simulink model "p3"  (R2014b)
settings: Solver=ode45  StartTime=0.0  StopTime=10  RelTol=1e-3
undefined symbols (not defined in the file): fdesignblkfcn, gcbh
settings Model: CovSFcnEnable=on  Creator=dhruv  LastModifiedBy=Kumar
settings OptimizationCC: UseDivisionForNetSlopeComputation=off  SimCompilerOptimization=off
settings DebuggingCC: SolverPrmCheckMsg=none  FrameProcessingCompatibilityMsg=error
settings RTWCC: RTWCompilerOptimization=off

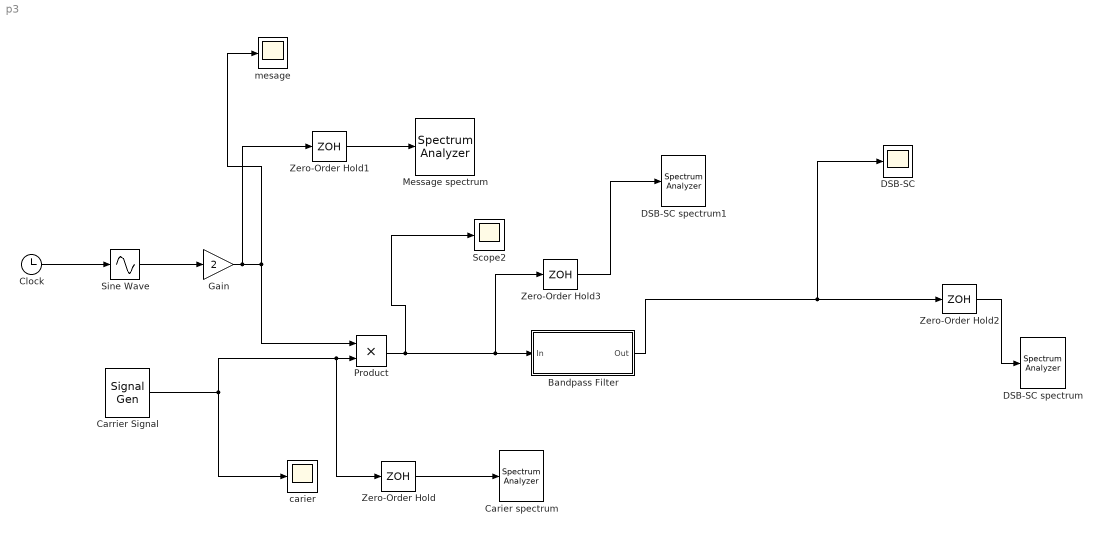
== system p3 ==
  Bandpass Filter : Subsystem  DialogController=fdesignblkfcn  InitFcn=fdesignblkfcn(gcbh, {'InitFcn'});  mask(Bandpass Filter){}
      mask help: Design a bandpass filter
      settings: CopyFcn=fdesignblkfcn(gcbh, {'CopyFcn'});
      mask Help: helpview(mapfilelocation('dsp'), 'dspbandpassfilter');
      mask Display: disp('Bandpass');
  Carier spectrum : SpectrumAnalyzer
  Carrier Signal : SignalGenerator  Frequency=5000
  Clock : Clock
  DSB-SC : Scope
      settings: SaveName=ScopeData4
  DSB-SC spectrum : SpectrumAnalyzer
  DSB-SC spectrum1 : SpectrumAnalyzer
  Gain : Gain  Gain=2
  Message spectrum : SpectrumAnalyzer
  Product : Product
  Scope2 : Scope
      settings: SaveName=ScopeData2
  Sine Wave : Sin  TimeSource=Use external signal  Frequency=2*pi*200  Phase=pi/2  SampleTime=1/4000
  Zero-Order Hold{,1..3} (4 alike) : ZeroOrderHold  SampleTime=1/30000
  carier : Scope
  mesage : Scope
      settings: TickLabels=on  TimeRange=0.05  SampleInput=on
  wires:
  Sine Wave/1 -> Gain/1
  Gain/1 -> Zero-Order Hold1/1, Product/1, mesage/1
  Zero-Order Hold1/1 -> Message spectrum/1
  Zero-Order Hold/1 -> Carier spectrum/1
  Carrier Signal/1 -> Zero-Order Hold/1, Product/2, carier/1
  Zero-Order Hold2/1 -> DSB-SC spectrum/1
  Clock/1 -> Sine Wave/1
  Product/1 -> Bandpass Filter/1(In), Zero-Order Hold3/1, Scope2/1
  Zero-Order Hold3/1 -> DSB-SC spectrum1/1
  Bandpass Filter/1(Out) -> DSB-SC/1, Zero-Order Hold2/1

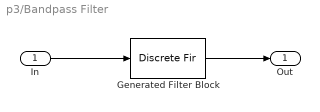
== system p3/Bandpass Filter ==
  In : Inport
  Generated Filter Block : DiscreteFir  Tag=BlockMethodSubSystem  Coefficients=[-4.2089415837660872e-05 -0.0014025699359127397 7.7506550936949734e-05 0.00057128919349381125 -9.8355641636346664e-05 -0.00066711051664750044 0.00015948550574925059 0.00075631980649035072 -0.00023183227068351514 -0.00083532589626739736 0.00031333464421453628 0.00089962011893319322 -0.00040054007469883838 -0.00094474087932631967 0.00048884052624121666 0.00096656259656608529 -0.00057259566206479542 -0.00096157278765519189 0.00064475645890059549 0.00092723279966929622 -0.00069727766749828413 -0.0008616969835593684 0.00072083712753834696 0.00076521221162942029 -0.00070602162712853241 -0.00063912529586439401 0.0006423406722035549 0.00048707943908900969 -0.00051996658042933281 -0.00031467504626851256 0.00032895848966047565 0.0001295769773692823 -5.9894635621539593e-05 5.8810688492332347e-05 -0.00029519389315708569 -0.00023886005831663434 0.00074344092220825773 0.00039759757148072599 -0.0012895192868593783 -0.00052014629591975385 0.0019357514526546135 0.00058978791876386971 -0.0026813185191843373 -0.00058969915231844752 0.0035228747461108953 0.00050249329706724723 -0.0044540262859193228 -0.00031132178874730622 0.005465652611708287 -2.0132267061769808e-08 -0.0065443773826657989 0.00044663404749908616 0.0076725252494337743 -0.0010421540717453555 -0.0088307194707965345 0.0017968251290740428 0.0099996125787013852 -0.0027156499402326666 -0.011152299522609547 0.0038070137168413377 0.012262744188026198 -0.0050656626714779083 -0.013305606273685999 0.0064903899880547249 0.014251503754626374 -0.0080706065000854827 -0.015074356999494659 0.0097933130913002066 0.015747812321655924 -0.011640237567196537 -0.016247827324636241 0.013589143049359908 0.016553020658669433 -0.015613894048028865 -0.016645297669244351 0.017684973480625265 0.01651066280843539 -0.01977035324422954 -0.016139584083822434 0.021835414838011533 0.015528220745682723 -0.02384516279173942 -0.014676806891530543 0.025763115190519308 0.013592405156089778 -0.027554730113670409 -0.012286369097904547 0.029185503080582365 0.010775414878743001 -0.030624623177874857 -0.0090826395283413134 0.03184344321980432 0.0072338476960973263 -0.032818065694990635 -0.0052594326922897321 0.03352876779753388 0.0031931316323640666 -0.033960794508747762 -0.0010707328789116388 0.034105765015016276 -0.0010707328789116388 -0.033960794508747762 0.0031931316323640666 0.03352876779753388 -0.0052594326922897321 -0.032818065694990635 0.0072338476960973263 0.03184344321980432 -0.0090826395283413134 -0.030624623177874857 0.010775414878743001 0.029185503080582365 -0.012286369097904547 -0.027554730113670409 0.013592405156089778 0.025763115190519308 -0.014676806891530543 -0.02384516279173942 0.015528220745682723 0.021835414838011533 -0.016139584083822434 -0.01977035324422954 0.01651066280843539 0.017684973480625265 -0.016645297669244351 -0.015613894048028865 0.016553020658669433 0.013589143049359908 -0.016247827324636241 -0.011640237567196537 0.015747812321655924 0.0097933130913002066 -0.015074356999494659 -0.0080706065000854827 0.014251503754626374 0.0064903899880547249 -0.013305606273685999 -0.0050656626714779083 0.012262744188026198 0.0038070137168413377 -0.011152299522609547 -0.0027156499402326666 0.0099996125787013852 0.0017968251290740428 -0.0088307194707965345 -0.0010421540717453555 0.0076725252494337743 0.00044663404749908616 -0.0065443773826657989 -2.0132267061769808e-08 0.005465652611708287 -0.00031132178874730622 -0.0044540262859193228 0.00050249329706724723 0.0035228747461108953 -0.00058969915231844752 -0.0026813185191843373 0.00058978791876386971 0.0019357514526546135 -0.00052014629591975385 -0.0012895192868593783 0.00039759757148072599 0.00074344092220825773 -0.00023886005831663434 -0.00029519389315708569 5.8810688492332347e-05 -5.9894635621539593e-05 0.0001295769773692823 0.00032895848966047565 -0.00031467504626851256 -0.00051996658042933281 0.00048707943908900969 0.0006423406722035549 -0.00063912529586439401 -0.00070602162712853241 0.00076521221162942029 0.00072083712753834696 -0.0008616969835593684 ...(+493 chars)]  InputProcessing=Columns as channels (frame based)
  Out : Outport
  wires:
  In/1 -> Generated Filter Block/1
  Generated Filter Block/1 -> Out/1
